simulink library "adeye_lib"  (R2019a)
settings: Solver=VariableStepAuto  StartTime=0.0  StopTime=10.0  RelTol=1e-3
undefined symbols (not defined in the file): AngularVelocity, Clock_, Data, Data_SL_Info, DiscIntNeverNeededParam, Encoding, Encoding_SL_Info, Header, Height, LinearAcceleration, Orientation, Pose, Step, Twist, Width
libraries: robotlib x47, $bdroot x46, simulink_extras x12, dspsrcs4 x6, dspindex x6, robotcorelib x2, aerolibutil x2, PreScanSimulinkLibrary x1
(part 4 of 4)

== system adeye_lib/Fault Injection Listener Lidar 1/If Action Subsystem ==
  In1 : Inport
  In2 : Inport  Port=2
  In3 : Inport  Port=3
  In4 : Inport  Port=4
  In5 : Inport  Port=5
  In6 : Inport  Port=6
  In7 : Inport  Port=7
  In8 : Inport  Port=8
  Action Port : ActionPort
  Out1 : Outport
  Out2 : Outport  Port=2
  Out3 : Outport  Port=3
  Out4 : Outport  Port=4
  Out5 : Outport  Port=5
  Out6 : Outport  Port=6
  Out7 : Outport  Port=7
  Out8 : Outport  Port=8
  wires:
  In1/1 -> Out1/1
  In2/1 -> Out2/1
  In3/1 -> Out3/1
  In4/1 -> Out4/1
  In5/1 -> Out5/1
  In6/1 -> Out6/1
  In7/1 -> Out7/1
  In8/1 -> Out8/1

== system adeye_lib/Fault Injection Listener Lidar 1/If Action Subsystem1 ==
  In1 : Inport
  In2 : Inport  Port=2
  In3 : Inport  Port=3
  In4 : Inport  Port=4
  In5 : Inport  Port=5
  In6 : Inport  Port=6
  In7 : Inport  Port=7
  In8 : Inport  Port=8
  Action Port : ActionPort
  Out1 : Outport
  Out2 : Outport  Port=2
  Out3 : Outport  Port=3
  Out4 : Outport  Port=4
  Out5 : Outport  Port=5
  Out6 : Outport  Port=6
  Out7 : Outport  Port=7
  Out8 : Outport  Port=8
  wires:
  In1/1 -> Out1/1
  In2/1 -> Out2/1
  In3/1 -> Out3/1
  In4/1 -> Out4/1
  In5/1 -> Out5/1
  In6/1 -> Out6/1
  In7/1 -> Out7/1
  In8/1 -> Out8/1

== system adeye_lib/Fault Injection Listener Lidar 2/If Action Subsystem ==
  In1 : Inport
  In2 : Inport  Port=2
  In3 : Inport  Port=3
  In4 : Inport  Port=4
  In5 : Inport  Port=5
  In6 : Inport  Port=6
  In7 : Inport  Port=7
  In8 : Inport  Port=8
  Action Port : ActionPort
  Out1 : Outport
  Out2 : Outport  Port=2
  Out3 : Outport  Port=3
  Out4 : Outport  Port=4
  Out5 : Outport  Port=5
  Out6 : Outport  Port=6
  Out7 : Outport  Port=7
  Out8 : Outport  Port=8
  wires:
  In1/1 -> Out1/1
  In2/1 -> Out2/1
  In3/1 -> Out3/1
  In4/1 -> Out4/1
  In5/1 -> Out5/1
  In6/1 -> Out6/1
  In7/1 -> Out7/1
  In8/1 -> Out8/1

== system adeye_lib/Fault Injection Listener Lidar 2/If Action Subsystem1 ==
  In1 : Inport
  In2 : Inport  Port=2
  In3 : Inport  Port=3
  In4 : Inport  Port=4
  In5 : Inport  Port=5
  In6 : Inport  Port=6
  In7 : Inport  Port=7
  In8 : Inport  Port=8
  Action Port : ActionPort
  Out1 : Outport
  Out2 : Outport  Port=2
  Out3 : Outport  Port=3
  Out4 : Outport  Port=4
  Out5 : Outport  Port=5
  Out6 : Outport  Port=6
  Out7 : Outport  Port=7
  Out8 : Outport  Port=8
  wires:
  In1/1 -> Out1/1
  In2/1 -> Out2/1
  In3/1 -> Out3/1
  In4/1 -> Out4/1
  In5/1 -> Out5/1
  In6/1 -> Out6/1
  In7/1 -> Out7/1
  In8/1 -> Out8/1

== system adeye_lib/Fault Injection Listener Lidar 3/If Action Subsystem ==
  In1 : Inport
  In2 : Inport  Port=2
  In3 : Inport  Port=3
  In4 : Inport  Port=4
  In5 : Inport  Port=5
  In6 : Inport  Port=6
  In7 : Inport  Port=7
  In8 : Inport  Port=8
  Action Port : ActionPort
  Out1 : Outport
  Out2 : Outport  Port=2
  Out3 : Outport  Port=3
  Out4 : Outport  Port=4
  Out5 : Outport  Port=5
  Out6 : Outport  Port=6
  Out7 : Outport  Port=7
  Out8 : Outport  Port=8
  wires:
  In1/1 -> Out1/1
  In2/1 -> Out2/1
  In3/1 -> Out3/1
  In4/1 -> Out4/1
  In5/1 -> Out5/1
  In6/1 -> Out6/1
  In7/1 -> Out7/1
  In8/1 -> Out8/1

== system adeye_lib/Fault Injection Listener Lidar 3/If Action Subsystem1 ==
  In1 : Inport
  In2 : Inport  Port=2
  In3 : Inport  Port=3
  In4 : Inport  Port=4
  In5 : Inport  Port=5
  In6 : Inport  Port=6
  In7 : Inport  Port=7
  In8 : Inport  Port=8
  Action Port : ActionPort
  Out1 : Outport
  Out2 : Outport  Port=2
  Out3 : Outport  Port=3
  Out4 : Outport  Port=4
  Out5 : Outport  Port=5
  Out6 : Outport  Port=6
  Out7 : Outport  Port=7
  Out8 : Outport  Port=8
  wires:
  In1/1 -> Out1/1
  In2/1 -> Out2/1
  In3/1 -> Out3/1
  In4/1 -> Out4/1
  In5/1 -> Out5/1
  In6/1 -> Out6/1
  In7/1 -> Out7/1
  In8/1 -> Out8/1

== system adeye_lib/Fault Injection Listener Lidar 4/If Action Subsystem ==
  In1 : Inport
  In2 : Inport  Port=2
  In3 : Inport  Port=3
  In4 : Inport  Port=4
  In5 : Inport  Port=5
  In6 : Inport  Port=6
  In7 : Inport  Port=7
  In8 : Inport  Port=8
  Action Port : ActionPort
  Out1 : Outport
  Out2 : Outport  Port=2
  Out3 : Outport  Port=3
  Out4 : Outport  Port=4
  Out5 : Outport  Port=5
  Out6 : Outport  Port=6
  Out7 : Outport  Port=7
  Out8 : Outport  Port=8
  wires:
  In1/1 -> Out1/1
  In2/1 -> Out2/1
  In3/1 -> Out3/1
  In4/1 -> Out4/1
  In5/1 -> Out5/1
  In6/1 -> Out6/1
  In7/1 -> Out7/1
  In8/1 -> Out8/1

== system adeye_lib/Fault Injection Listener Lidar 4/If Action Subsystem1 ==
  In1 : Inport
  In2 : Inport  Port=2
  In3 : Inport  Port=3
  In4 : Inport  Port=4
  In5 : Inport  Port=5
  In6 : Inport  Port=6
  In7 : Inport  Port=7
  In8 : Inport  Port=8
  Action Port : ActionPort
  Out1 : Outport
  Out2 : Outport  Port=2
  Out3 : Outport  Port=3
  Out4 : Outport  Port=4
  Out5 : Outport  Port=5
  Out6 : Outport  Port=6
  Out7 : Outport  Port=7
  Out8 : Outport  Port=8
  wires:
  In1/1 -> Out1/1
  In2/1 -> Out2/1
  In3/1 -> Out3/1
  In4/1 -> Out4/1
  In5/1 -> Out5/1
  In6/1 -> Out6/1
  In7/1 -> Out7/1
  In8/1 -> Out8/1

== system adeye_lib/Fault Injection Listener Radar/If Action Subsystem ==
  In1 : Inport
  In2 : Inport  Port=2
  In3 : Inport  Port=3
  In4 : Inport  Port=4
  Action Port : ActionPort  ActionPortLabel=if(u1 > 0)
  Out1 : Outport
  Out2 : Outport  Port=2
  Out3 : Outport  Port=3
  Out4 : Outport  Port=4
  wires:
  In1/1 -> Out1/1
  In2/1 -> Out2/1
  In3/1 -> Out3/1
  In4/1 -> Out4/1

== system adeye_lib/Fault Injection Listener Radar/If Action Subsystem1 ==
  In1 : Inport
  In2 : Inport  Port=2
  In3 : Inport  Port=3
  In4 : Inport  Port=4
  Action Port : ActionPort  ActionPortLabel=else
  Out1 : Outport
  Out2 : Outport  Port=2
  Out3 : Outport  Port=3
  Out4 : Outport  Port=4
  wires:
  In1/1 -> Out1/1
  In2/1 -> Out2/1
  In3/1 -> Out3/1
  In4/1 -> Out4/1

== system adeye_lib/Fault Injection Listener TL Camera/If Action Subsystem ==
  In1 : Inport
  In2 : Inport  Port=2
  In3 : Inport  Port=3
  In4 : Inport  Port=4
  In5 : Inport  Port=5
  In6 : Inport  Port=6
  In7 : Inport  Port=7
  In8 : Inport  Port=8
  Action Port : ActionPort
  Out1 : Outport
  Out2 : Outport  Port=2
  Out3 : Outport  Port=3
  Out4 : Outport  Port=4
  Out5 : Outport  Port=5
  Out6 : Outport  Port=6
  Out7 : Outport  Port=7
  Out8 : Outport  Port=8
  wires:
  In1/1 -> Out1/1
  In2/1 -> Out2/1
  In3/1 -> Out3/1
  In4/1 -> Out4/1
  In5/1 -> Out5/1
  In6/1 -> Out6/1
  In7/1 -> Out7/1
  In8/1 -> Out8/1

== system adeye_lib/Fault Injection Listener TL Camera/If Action Subsystem1 ==
  In1 : Inport
  In2 : Inport  Port=2
  In3 : Inport  Port=3
  In4 : Inport  Port=4
  In5 : Inport  Port=5
  In6 : Inport  Port=6
  In7 : Inport  Port=7
  In8 : Inport  Port=8
  Action Port : ActionPort
  Out1 : Outport
  Out2 : Outport  Port=2
  Out3 : Outport  Port=3
  Out4 : Outport  Port=4
  Out5 : Outport  Port=5
  Out6 : Outport  Port=6
  Out7 : Outport  Port=7
  Out8 : Outport  Port=8
  wires:
  In1/1 -> Out1/1
  In2/1 -> Out2/1
  In3/1 -> Out3/1
  In4/1 -> Out4/1
  In5/1 -> Out5/1
  In6/1 -> Out6/1
  In7/1 -> Out7/1
  In8/1 -> Out8/1

== system adeye_lib/Fault Injection Radar/If Action Subsystem ==
  In1 : Inport
  In2 : Inport  Port=2
  In3 : Inport  Port=3
  In4 : Inport  Port=4
  Action Port : ActionPort
  Out1 : Outport
  Out2 : Outport  Port=2
  Out3 : Outport  Port=3
  Out4 : Outport  Port=4
  wires:
  In4/1 -> Out4/1
  In3/1 -> Out3/1
  In2/1 -> Out2/1
  In1/1 -> Out1/1

== system adeye_lib/Fault Injection Radar/If Action Subsystem1 ==
  range : Inport
  theta : Inport  Port=2
  phi : Inport  Port=3
  In4 : Inport  Port=4
  range_variance : Inport  Port=5
  theta_variance : Inport  Port=6
  phi_variance : Inport  Port=7
  Action Port : ActionPort
  Add : Sum
  Add1 : Sum
  Add2 : Sum
  Product1 : Product
  Product2 : Product
  Product3 : Product
  Random Number : RandomNumber  Seed=1:1:n  SampleTime=0.05
  Random Number1 : RandomNumber  Seed=n+1:1:2*n  SampleTime=0.05
  Random Number2 : RandomNumber  Seed=2*n+1:1:3*n  SampleTime=0.05
  Sqrt : Sqrt  SaturateOnIntegerOverflow=on
  Sqrt1 : Sqrt  SaturateOnIntegerOverflow=on
  Sqrt2 : Sqrt  SaturateOnIntegerOverflow=on
  Out1 : Outport
  Out2 : Outport  Port=2
  Out3 : Outport  Port=3
  Out4 : Outport  Port=4
  wires:
  phi/1 -> Add2/2
  Add/1 -> Out2/1
  Add1/1 -> Out1/1
  In4/1 -> Out4/1
  theta/1 -> Add/2
  range/1 -> Add1/2
  Add2/1 -> Out3/1
  range_variance/1 -> Sqrt/1
  Sqrt/1 -> Product3/1
  Random Number/1 -> Product3/2
  Product3/1 -> Add1/1
  Sqrt1/1 -> Product1/1
  theta_variance/1 -> Sqrt1/1
  Random Number1/1 -> Product1/2
  Product1/1 -> Add/1
  phi_variance/1 -> Sqrt2/1
  Sqrt2/1 -> Product2/1
  Product2/1 -> Add2/1
  Random Number2/1 -> Product2/2

== system adeye_lib/Lidar Adapter/Rotate over Z ==
  In1 : Inport
  In2 : Inport  Port=2
  In3 : Inport  Port=3
  Add : Sum  Inputs=+-
  Add1 : Sum
  Degrees to Radians1 : simulink_extras/Transformations/Degrees to Radians
  Product{,1..3} (4 alike) : Product
  Trigonometric Function : Trigonometry
  Trigonometric Function1 : Trigonometry  Operator=cos
  Out1 : Outport
  Out2 : Outport  Port=2
  wires:
  Add/1 -> Out1/1
  In1/1 -> Degrees to Radians1/1
  In3/1 -> Product1/2, Product3/2
  Product2/1 -> Add1/1
  Product1/1 -> Add/2
  Add1/1 -> Out2/1
  Product3/1 -> Add1/2
  Degrees to Radians1/1 -> Trigonometric Function/1, Trigonometric Function1/1
  Trigonometric Function1/1 -> Product3/1, Product/1
  Trigonometric Function/1 -> Product1/1, Product2/1
  Product/1 -> Add/1
  In2/1 -> Product2/2, Product/2

== system adeye_lib/Lidar Adapter/Spherical to cartesian ==
  In1 : Inport
  In2 : Inport  Port=2
  In3 : Inport  Port=3
  Constant : Constant  Value=-1  OutDataTypeStr=Inherit: Inherit via back propagation
  Product : Product
  Product1 : Product  Inputs=3
  Product2 : Product  Inputs=3
  Product3 : Product
  Trigonometric Function : Trigonometry  Operator=cos
  Trigonometric Function1 : Trigonometry
  Trigonometric Function2 : Trigonometry  Operator=cos
  Trigonometric Function3 : Trigonometry
  Out1 : Outport
  Out2 : Outport  Port=2
  Out3 : Outport  Port=3
  wires:
  In2/1 -> Trigonometric Function2/1, Trigonometric Function3/1
  In3/1 -> Trigonometric Function/1, Trigonometric Function1/1
  Product3/1 -> Out2/1
  Constant/1 -> Product3/2
  Trigonometric Function/1 -> Product2/2, Product1/2
  Trigonometric Function1/1 -> Product/2
  Trigonometric Function2/1 -> Product1/3
  Trigonometric Function3/1 -> Product2/3
  Product2/1 -> Product3/1
  Product1/1 -> Out1/1
  Product/1 -> Out3/1
  In1/1 -> Product1/1, Product/1, Product2/1

== system adeye_lib/ROS Send Simulink State/If Action Subsystem ==
  In1 : Inport
  In2 : Inport  Port=2
  In3 : Inport  Port=3
  In4 : Inport  Port=4
  In5 : Inport  Port=5
  In6 : Inport  Port=6
  In7 : Inport  Port=7
  In8 : Inport  Port=8
  In9 : Inport  Port=9
  In10 : Inport  Port=10
  In11 : Inport  Port=11
  Action Port : ActionPort  ActionPortLabel=if(u1 > 0.5)
  Out1 : Outport
  Out2 : Outport  Port=2
  Out3 : Outport  Port=3
  Out4 : Outport  Port=4
  Out5 : Outport  Port=5
  Out6 : Outport  Port=6
  Out7 : Outport  Port=7
  Out8 : Outport  Port=8
  Out9 : Outport  Port=9
  Out10 : Outport  Port=10
  Out11 : Outport  Port=11
  wires:
  In1/1 -> Out1/1
  In2/1 -> Out2/1
  In3/1 -> Out3/1
  In4/1 -> Out4/1
  In5/1 -> Out5/1
  In6/1 -> Out6/1
  In7/1 -> Out7/1
  In8/1 -> Out8/1
  In9/1 -> Out9/1
  In10/1 -> Out10/1
  In11/1 -> Out11/1

== system adeye_lib/ROS Send Simulink State/If Action Subsystem2 ==
  Action Port : ActionPort  ActionPortLabel=else
  Detection : Constant
  FakeLocalization : Constant
  Localization : Constant  Value=0
  Map : Constant
  MissionPlanning : Constant
  MotionPlanning : Constant
  Recording : Constant
  Rviz : Constant
  Sensing : Constant
  Ssmp : Constant
  Switch : Constant
  Out1 : Outport  InitialOutput=[0]
  Out2 : Outport  Port=2  InitialOutput=[0]
  Out3 : Outport  Port=3  InitialOutput=[0]
  Out4 : Outport  Port=4  InitialOutput=[0]
  Out5 : Outport  Port=5  InitialOutput=[0]
  Out6 : Outport  Port=6  InitialOutput=[0]
  Out7 : Outport  Port=7  InitialOutput=[0]
  Out8 : Outport  Port=8  InitialOutput=[0]
  Out9 : Outport  Port=9  InitialOutput=[0]
  Out10 : Outport  Port=10  InitialOutput=[0]
  Out11 : Outport  Port=11  InitialOutput=[0]
  wires:
  Recording/1 -> Out1/1
  Map/1 -> Out2/1
  Sensing/1 -> Out3/1
  Localization/1 -> Out4/1
  FakeLocalization/1 -> Out5/1
  Detection/1 -> Out6/1
  MissionPlanning/1 -> Out7/1
  MotionPlanning/1 -> Out8/1
  Switch/1 -> Out9/1
  Ssmp/1 -> Out10/1
  Rviz/1 -> Out11/1

== system adeye_lib/Subsystem1/Subsystem ==
  note: Current
  note: Desired
  In1 : Inport
  In2 : Inport  Port=2
  Acceleration bound (m/s^2) : Constant  Value=3
  Clock : Clock
  If : If  NumInputs=2  IfExpression=u1 > u2  ElseIfExpressions=u1 > -u2
  If Action Subsystem : Subsystem  TreatAsAtomicUnit=on
  If Action Subsystem1 : Subsystem  TreatAsAtomicUnit=on
  If Action Subsystem2 : Subsystem  TreatAsAtomicUnit=on
  Memory : Memory
  Merge : Merge  Inputs=3
  Product : Product
  Subtract : Sum  Inputs=-+
  Subtract1 : Sum  Inputs=+-
  Out1 : Outport
  wires:
  Memory/1 -> Subtract1/2
  Clock/1 -> Subtract1/1, Memory/1
  Acceleration bound (m/s^2)/1 -> Product/2
  Product/1 -> If Action Subsystem/2(In2), If Action Subsystem1/2(In2), If/2
  Subtract1/1 -> Product/1
  Subtract/1 -> If/1
  In2/1 -> If Action Subsystem2/1(In1), Subtract/2
  In1/1 -> Subtract/1, If Action Subsystem/1(In1), If Action Subsystem1/1(In1)
  If Action Subsystem1/1(Out1) -> Merge/3
  If/1 -> If Action Subsystem/Action
  If/2 -> If Action Subsystem2/Action
  If Action Subsystem2/1(Out1) -> Merge/2
  Merge/1 -> Out1/1
  If/3 -> If Action Subsystem1/Action
  If Action Subsystem/1(Out1) -> Merge/1

== system adeye_lib/radarDetections/Spherical to cartesian ==
  In1 : Inport
  In2 : Inport  Port=2
  In3 : Inport  Port=3
  Constant : Constant  Value=-1  OutDataTypeStr=Inherit: Inherit via back propagation
  Product : Product
  Product1 : Product  Inputs=3
  Product2 : Product  Inputs=3
  Product3 : Product
  Trigonometric Function : Trigonometry  Operator=cos
  Trigonometric Function1 : Trigonometry
  Trigonometric Function2 : Trigonometry  Operator=cos
  Trigonometric Function3 : Trigonometry
  Out1 : Outport
  Out2 : Outport  Port=2
  Out3 : Outport  Port=3
  wires:
  In2/1 -> Trigonometric Function2/1, Trigonometric Function3/1
  In3/1 -> Trigonometric Function/1, Trigonometric Function1/1
  Product3/1 -> Out2/1
  Constant/1 -> Product3/2
  Trigonometric Function/1 -> Product2/2, Product1/2
  Trigonometric Function1/1 -> Product/2
  Trigonometric Function2/1 -> Product1/3
  Trigonometric Function3/1 -> Product2/3
  Product2/1 -> Product3/1
  Product1/1 -> Out1/1
  Product/1 -> Out3/1
  In1/1 -> Product1/1, Product/1, Product2/1

== system adeye_lib/Subsystem1/Subsystem/If Action Subsystem ==
  In1 : Inport
  In2 : Inport  Port=2
  Action Port : ActionPort
  Add : Sum
  Out1 : Outport
  wires:
  Add/1 -> Out1/1
  In1/1 -> Add/1
  In2/1 -> Add/2

== system adeye_lib/Subsystem1/Subsystem/If Action Subsystem1 ==
  In1 : Inport
  In2 : Inport  Port=2
  Action Port : ActionPort
  Add : Sum  Inputs=+-
  Out1 : Outport
  wires:
  Add/1 -> Out1/1
  In2/1 -> Add/2
  In1/1 -> Add/1

== system adeye_lib/Subsystem1/Subsystem/If Action Subsystem2 ==
  In1 : Inport
  Action Port : ActionPort
  Out1 : Outport
  wires:
  In1/1 -> Out1/1

== matlab function adeye_lib/ROS Send Camera TL/VECTORES ==
  data: imgR input; data output; imgG input; imgB input
function data = fcn(imgR, imgG, imgB)
L=length(imgR);
data=zeros(1,L*3);
data(1:3:end)=imgR;
data(2:3:end)=imgG;
data(3:3:end)=imgB;

== matlab function adeye_lib/pcd_writer/MATLAB Function ==
  data: u input

function fcn(u)
Path_to_Data_Folder = "..\Pointcloud_Files\";
coder.extrinsic('clock')
coder.extrinsic('num2str')
coder.extrinsic('strcat')
coder.extrinsic('pcwrite')
coder.extrinsic('pointCloud')
xyzPoints=u(:,1:3);
Intensities=u(:,4);
ptCloud=pointCloud(xyzPoints,"Intensity",Intensities);

c=clock;
filename=strcat(Path_to_Data_Folder,"pcd_",num2str(fix(c(4))),"_",num2str(fix(c(5))),"_",num2str(fix(1000*c(6))),".pcd");
pcwrite(ptCloud,filename);
